simulink model "Associativity_16_taps"  (R2021a)
settings: Solver=VariableStepAuto  StartTime=0.0  StopTime=4000  RelTol=1e-3
undefined symbols (not defined in the file): variable_step_size_calc, variable_step_size_calc_1, x1
libraries: dspsrcs4 x4
settings Model: Creator=HP  LastModifiedBy=HP

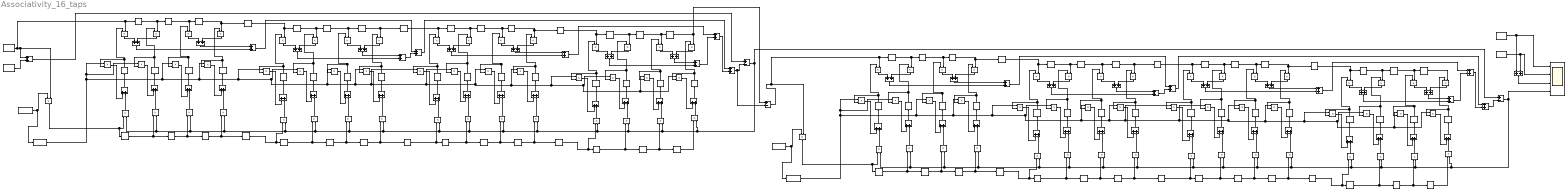
== system Associativity_16_taps ==
  Add{1..31,33..57,59..62,64..67} (64 alike) : Sum
  Add32 : Sum  Inputs=+-
  Add58 : Sum  Inputs=+-
  Add63 : Sum  Inputs=+-
  Delay{,1..91} (92 alike) : Delay  DelayLength=1  InitialCondition=0
  ECG SIGNAL : dspsrcs4/Signal From Workspace  X=m1  Ts=1  nsamps=1  OutputAfterFinalValue=Setting to zero  ignoreOrWarnInputAndFrameLengths=off  OutputFrames=off
  Interpreted MATLAB Function : MATLABFcn  MATLABFcn=LeakyFactorCalc
  Interpreted MATLAB Function1 : MATLABFcn  MATLABFcn=variable_step_size_calc(x1)
  Interpreted MATLAB Function2 : MATLABFcn  MATLABFcn=LeakyFactorCalc
  Interpreted MATLAB Function3 : MATLABFcn  MATLABFcn=variable_step_size_calc_1(x1)
  PLI NOISE : dspsrcs4/Signal From Workspace  X=x1  Ts=1  nsamps=1  OutputAfterFinalValue=Setting to zero  ignoreOrWarnInputAndFrameLengths=off  OutputFrames=off
  PLI NOISE1 : dspsrcs4/Signal From Workspace  X=m1  Ts=1  nsamps=1  OutputAfterFinalValue=Setting to zero  ignoreOrWarnInputAndFrameLengths=off  OutputFrames=off
  PLI NOISE2 : dspsrcs4/Signal From Workspace  X=x1  Ts=1  nsamps=1  OutputAfterFinalValue=Setting to zero  ignoreOrWarnInputAndFrameLengths=off  OutputFrames=off
  Product{,1..97} (98 alike) : Product
  Time Scope : Scope  NumInputPorts=4
  wires:
  Delay26/1 -> Product33/2, Add63/1
  Delay37/1 -> Product25/1, Product35/2
  Product38/1 -> Add27/1
  Product12/1 -> Add10/1
  Product22/1 -> Add10/2
  Add28/1 -> Delay40/1
  Interpreted MATLAB Function1/1 -> Interpreted MATLAB Function/1, Product8/1
  Add11/1 -> Delay15/1
  Product14/1 -> Add11/1
  Product20/1 -> Add5/1
  Delay32/1 -> Delay33/1, Product41/1
  Product5/1 -> Add4/2
  Delay2/1 -> Delay21/1, Product3/2
  Add3/1 -> Delay3/1
  Delay9/1 -> Delay20/1, Product7/1
  Delay1/1 -> Product2/2, Delay2/1
  Delay7/1 -> Delay8/1, Product5/1
  Add4/1 -> Delay4/1
  Product35/1 -> Add25/1
  Add27/1 -> Delay39/1
  Delay18/1 -> Delay19/1, Product23/1
  Product44/1 -> Add25/2
  Delay21/1 -> Product9/2, Delay10/1
  Product23/1 -> Add11/2
  Product17/1 -> Add9/2
  Product6/1 -> Add5/2
  Delay22/1 -> Product26/2, Delay23/1
  Add6/1 -> Delay6/1
  Add7/1 -> Add32/1
  Delay11/1 -> Product13/2, Delay12/1
  Delay43/1 -> Delay35/1, Product47/1
  Delay36/1 -> Product48/2, Delay24/1
  Add26/1 -> Delay38/1
  Delay40/1 -> Product39/2, Product43/1
  Product18/1 -> Add3/1
  Delay3/1 -> Product/1, Product18/2
  Delay35/1 -> Product34/1, Delay31/1
  Delay15/1 -> Product14/2, Product13/1
  Product36/1 -> Add26/1
  Product28/1 -> Add30/1
  Delay25/1 -> Product30/2, Delay26/1
  Delay39/1 -> Product38/2, Product37/1
  Delay33/1 -> Product42/1
  Product29/1 -> Add18/1
  Delay19/1 -> Product24/1, Delay44/1
  Delay4/1 -> Product19/2, Product1/1
  Add12/1 -> Delay16/1
  Add30/1 -> Delay27/1
  Add18/1 -> Delay28/1
  Delay5/1 -> Product20/2, Product2/1
  Product45/1 -> Add26/2
  Product7/1 -> Add6/2
  Add25/1 -> Delay37/1
  Delay10/1 -> Product10/2, Delay11/1
  Product47/1 -> Add28/2
  Product32/1 -> Add20/1
  Product40/1 -> Add18/2
  PLI NOISE/1 -> Product/2, Delay/1, Product8/2, Add7/1
  Add10/1 -> Delay14/1
  Interpreted MATLAB Function/1 -> Product20/1, Product21/1, Product14/1, Product39/1, Product31/1, Product32/1, Product29/1, Product28/1, Product38/1, Product36/1, Product35/1, Product15/1, Product12/1, Product11/1, Product19/1, Product18/1
  Delay44/1 -> Product44/1, Delay41/1
  Delay14/1 -> Product12/2, Product10/1
  Product11/1 -> Add9/1
  Product15/1 -> Add12/1
  Delay34/1 -> Delay36/1, Product43/2
  Add5/1 -> Delay5/1
  Delay17/1 -> Delay18/1, Product22/1
  Delay16/1 -> Product15/2, Product16/1
  Delay38/1 -> Product36/2, Product26/1
  Product4/1 -> Add3/2
  Product42/1 -> Add20/2
  Delay41/1 -> Delay42/1, Product45/1
  Delay13/1 -> Product9/1, Product11/2
  Delay28/1 -> Product29/2, Product27/1
  Delay24/1 -> Product27/2, Delay25/1
  Delay23/1 -> Product37/2, Delay34/1
  Delay27/1 -> Product48/1, Product28/2
  Product46/1 -> Add27/2
  Product19/1 -> Add4/1
  Product39/1 -> Add28/1
  Delay6/1 -> Product21/2, Product3/1
  Delay8/1 -> Delay9/1, Product6/1
  Product24/1 -> Add12/2
  Delay12/1 -> Delay45/1, Product16/2
  Add19/1 -> Delay29/1
  Delay31/1 -> Delay32/1, Product40/1
  Product31/1 -> Add19/1
  Delay45/1 -> Product25/2, Delay22/1
  Product21/1 -> Add6/1
  Delay42/1 -> Delay43/1, Product46/1
  Add20/1 -> Delay30/1
  Delay20/1 -> Product17/1, Delay17/1
  Product41/1 -> Add19/2
  ECG SIGNAL/1 -> Add7/2
  Delay30/1 -> Product32/2, Product33/1
  Add9/1 -> Delay13/1
  Delay29/1 -> Product31/2, Product30/1
  Delay/1 -> Product1/2, Delay1/1
  Product8/1 -> Product4/1, Delay7/1
  Product34/1 -> Add30/2
  Product/1 -> Add1/1
  Product1/1 -> Add1/2
  Product2/1 -> Add67/1
  Product3/1 -> Add67/2
  Add67/1 -> Add13/1
  Add1/1 -> Add13/2
  Product9/1 -> Add2/1
  Product10/1 -> Add2/2
  Product13/1 -> Add8/1
  Product16/1 -> Add8/2
  Add8/1 -> Add15/1
  Add2/1 -> Add15/2
  Product25/1 -> Add14/1
  Product26/1 -> Add14/2
  Product37/1 -> Add16/1
  Product43/1 -> Add16/2
  Add16/1 -> Add21/1
  Add14/1 -> Add21/2
  Product48/1 -> Add17/1
  Product27/1 -> Add17/2
  Product30/1 -> Add22/1
  Product33/1 -> Add22/2
  Add22/1 -> Add23/1
  Add17/1 -> Add23/2
  Add15/1 -> Add24/2
  Add13/1 -> Add24/1
  Add21/1 -> Add29/1
  Add23/1 -> Add29/2
  Add24/1 -> Add31/1
  Add29/1 -> Add31/2
  Add31/1 -> Add63/2, Add32/2
  Product51/1 -> Add44/2
  Product68/1 -> Add38/2
  Add39/1 -> Add49/2
  Product67/1 -> Add38/1
  Product57/1 -> Add64/2
  Product90/1 -> Add52/2
  Delay66/1 -> Product92/1, Product70/2
  Delay62/1 -> Product80/2, Delay74/1
  Delay67/1 -> Product71/2, Product69/1
  Delay51/1 -> Product97/1, Product52/2
  Delay82/1 -> Delay83/1, Product89/1
  Product69/1 -> Add41/2
  Product83/1 -> Add55/2
  Product86/1 -> Add45/2
  Add57/1 -> Add58/2
  Delay68/1 -> Product74/2, Product73/1
  Add65/1 -> Delay51/1
  Delay70/1 -> Product75/2, Product76/1
  Add45/1 -> Delay70/1
  Delay83/1 -> Delay84/1, Product90/1
  Product63/1 -> Add61/1
  Delay86/1 -> Product67/2, Delay61/1
  Add58/1 -> Product86/2, Product85/2, Product84/2, Product77/2, Product91/2, Product90/2, Product89/2, Product66/2, Product65/2, Product64/2, Product58/2, Product95/2, Product94/2, Product93/2, Product83/2, Product88/2, Time Scope/4
  Product74/1 -> Add43/1
  Product80/1 -> Add40/1
  Add47/1 -> Add48/1
  Add44/1 -> Add39/2
  Product61/1 -> Add62/1
  Delay50/1 -> Delay86/1, Product57/2
  Add43/1 -> Delay68/1
  Delay90/1 -> Delay91/1, Product94/1
  Add40/1 -> Add46/1
  Product60/1 -> Add59/1
  Product82/1 -> Add53/1
  Delay77/1 -> Product67/1, Product78/2
  Delay65/1 -> Product76/2
  Product50/1 -> Add33/2
  Add62/1 -> Add37/1
  Add49/1 -> Add57/1
  Product71/1 -> Add42/1
  Product73/1 -> Add47/1
  Delay73/1 -> Product86/1
  Product87/1 -> Add40/2
  Product88/1 -> Add50/2
  Delay56/1 -> Delay57/1, Product65/1
  Add52/1 -> Delay79/1
  Delay89/1 -> Delay90/1, Product93/1
  Add59/1 -> Delay80/1
  Delay91/1 -> Delay59/1, Product95/1
  Add55/1 -> Delay69/1
  Add35/1 -> Delay53/1
  Delay58/1 -> Delay60/1, Product72/2
  Add46/1 -> Add54/1
  Interpreted MATLAB Function3/1 -> Interpreted MATLAB Function2/1, Product96/1
  Add38/1 -> Add46/2
  Delay63/1 -> Product69/2, Delay64/1
  Add53/1 -> Delay81/1
  Product72/1 -> Add62/2
  Product64/1 -> Add34/2
  Product53/1 -> Add34/1
  Delay53/1 -> Product55/2, Product54/1
  Delay75/1 -> Product77/1, Delay71/1
  Add41/1 -> Add48/2
  Product79/1 -> Add51/1
  Add33/1 -> Add37/2
  Product59/1 -> Add55/1
  Delay59/1 -> Product58/1, Delay55/1
  Delay69/1 -> Product49/1, Product59/2
  Delay81/1 -> Product82/2, Product87/1
  Product66/1 -> Add36/2
  Product62/1 -> Add60/1
  Delay84/1 -> Delay75/1, Product91/1
  Delay76/1 -> Product92/2, Delay63/1
  Delay49/1 -> Product54/2, Delay50/1
  Add32/1 -> Product42/2, Product41/2, Product40/2, Product34/2, Product47/2, Product46/2, Product45/2, Product24/2, Product23/2, Product22/2, Product17/2, Product7/2, Product6/2, Product5/2, Product4/2, Product44/2, Add58/1
  Add61/1 -> Delay88/1
  Product94/1 -> Add60/2
  Delay61/1 -> Product68/2, Delay62/1
  Product65/1 -> Add35/2
  Delay60/1 -> Product97/2, Delay48/1
  Product58/1 -> Add65/2
  Delay78/1 -> Product79/2, Product68/1
  Product85/1 -> Add43/2
  Delay55/1 -> Delay56/1, Product64/1
  Delay54/1 -> Product56/2, Product57/1
  Add54/1 -> Add57/2
  Add60/1 -> Delay87/1
  Delay74/1 -> Delay76/1, Product87/2
  Product56/1 -> Add36/1
  Delay52/1 -> Product53/2, Product51/1
  Add42/1 -> Delay67/1
  Add56/1 -> Delay66/1
  Delay80/1 -> Product60/2, Product50/1
  Delay79/1 -> Product81/2, Product80/1
  Add51/1 -> Delay78/1
  Product70/1 -> Add56/1
  Product95/1 -> Add61/2
  Product89/1 -> Add51/2
  Delay87/1 -> Product62/2, Product61/1
  Product77/1 -> Add56/2
  Product54/1 -> Add64/1
  Product97/1 -> Add44/1
  Delay48/1 -> Product51/2, Delay49/1
  Product55/1 -> Add35/1
  Add50/1 -> Delay77/1
  Add48/1 -> Add54/2
  Product52/1 -> Add65/1
  Product49/1 -> Add33/1
  Delay72/1 -> Delay73/1, Product85/1
  Delay57/1 -> Product66/1, Delay85/1
  Delay88/1 -> Product63/2, Product72/1
  Product81/1 -> Add52/1
  Add37/1 -> Add49/1
  Add64/1 -> Add39/1
  Delay47/1 -> Product61/2, Delay58/1
  Product91/1 -> Add53/2
  Product93/1 -> Add59/2
  Product76/1 -> Add47/2
  Add34/1 -> Delay52/1
  Add63/1 -> Product49/2, Delay46/1, Product96/2
  Product96/1 -> Product83/1, Delay89/1
  Delay71/1 -> Delay72/1, Product84/1
  Product92/1 -> Add41/1
  Interpreted MATLAB Function2/1 -> Product62/1, Product63/1, Product55/1, Product82/1, Product74/1, Product75/1, Product71/1, Product70/1, Product81/1, Product79/1, Product78/1, Product56/1, Product53/1, Product52/1, Product60/1, Product59/1
  Delay64/1 -> Product73/2, Delay65/1
  Delay85/1 -> Product88/1, Delay82/1
  Product75/1 -> Add45/1
  Delay46/1 -> Product50/2, Delay47/1
  Add36/1 -> Delay54/1
  Product84/1 -> Add42/2
  Product78/1 -> Add50/1
  PLI NOISE1/1 -> Add66/1, Time Scope/1
  PLI NOISE2/1 -> Add66/2, Time Scope/2
  Add66/1 -> Time Scope/3
